simulink model "pcc_backstepping_piston_velocity_loop"  (R2021a)
settings: Solver=VariableStepAuto  StartTime=0.0  StopTime=70  MaxStep=0.001  RelTol=1e-3
undefined symbols (not defined in the file): l, q_eq, tol_q_stable
libraries: simulink_extras x4, simulink x3, pid_lib x1
settings Model: PauseTimes=0  Creator=maximilianstoelzle  LastModifiedBy=mstolzle
settings RTWCC: BuildConfiguration=Faster Runs

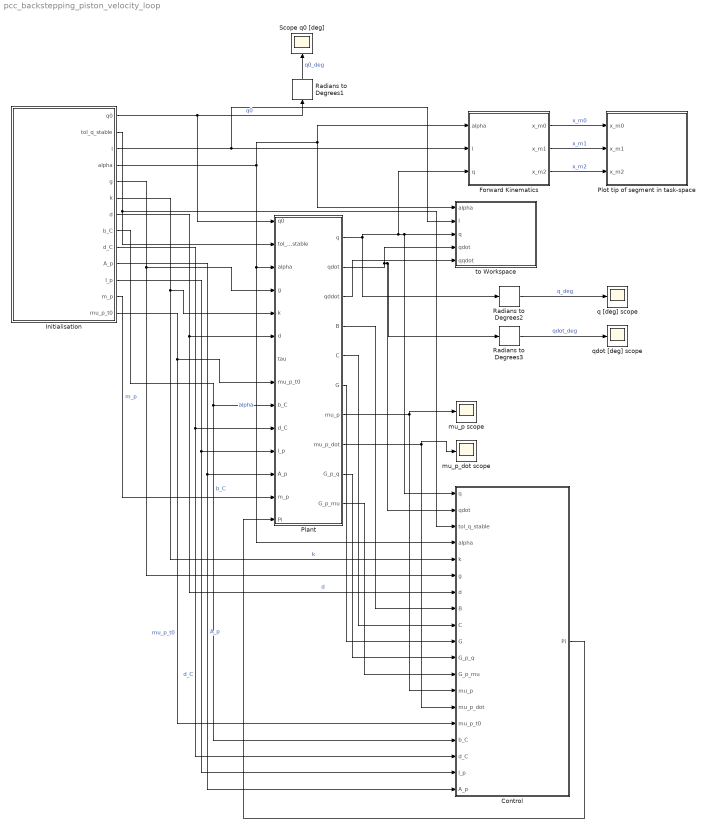
== system pcc_backstepping_piston_velocity_loop ==
  Control : Subsystem
  Forward Kinematics : MATLAB Function  TreatAsAtomicUnit=on
  Initialisation : Subsystem
  Plant : Subsystem
  Plot tip of segment in task-space : Subsystem
  Radians to Degrees1 : simulink_extras/Transformations/Radians to Degrees
  Radians to Degrees2 : simulink_extras/Transformations/Radians to Degrees
  Radians to Degrees3 : simulink_extras/Transformations/Radians to Degrees
  Scope q0 [deg] : Scope
  mu_p scope : Scope
  mu_p_dot scope : Scope
  q [deg] scope : Scope
  qdot [deg] scope : Scope
  to Workspace : Subsystem
  wires:
  Initialisation/12(m_p) -> Plant/13(m_p)  "m_p"
  Plant/5(C) -> Control/9(C)
  Initialisation/13(mu_p_t0) -> Control/15(mu_p_t0), Plant/8(mu_p_t0)  "mu_p_t0"
  Plant/10(G_p_mu) -> Control/12(G_p_mu)
  Initialisation/6(k) -> Control/5(k), Plant/5(k)  "k"
  Plant/8(mu_p_dot) -> mu_p_dot scope/1, Control/14(mu_p_dot)
  Plant/9(G_p_q) -> Control/11(G_p_q)
  Control/1(Pi) -> Plant/14(Pi)
  Radians to Degrees1/1 -> Scope q0 [deg]/1  "q0_deg"
  Plant/6(G) -> Control/10(G)
  Plant/4(B) -> Control/8(B)
  Initialisation/5(g) -> Control/6(g), Plant/4(g)
  Plant/3(qddot) -> to Workspace/5(qqdot)
  Radians to Degrees3/1 -> qdot [deg] scope/1  "qdot_deg"
  Forward Kinematics/3(x_m2) -> Plot tip of segment in task-space/3(x_m2)  "x_m2"
  Forward Kinematics/2(x_m1) -> Plot tip of segment in task-space/2(x_m1)  "x_m1"
  Forward Kinematics/1(x_m0) -> Plot tip of segment in task-space/1(x_m0)  "x_m0"
  Radians to Degrees2/1 -> q [deg] scope/1  "q_deg"
  Plant/7(mu_p) -> mu_p scope/1, Control/13(mu_p)
  Initialisation/11(l_p) -> Control/18(l_p), Plant/11(l_p)
  Initialisation/8(b_C) -> Control/16(b_C), Plant/9(b_C)  "b_C"
  Initialisation/9(d_C) -> Control/17(d_C), Plant/10(d_C)  "d_C"
  Initialisation/10(A_p) -> Control/19(A_p), Plant/12(A_p)  "A_p"
  Initialisation/1(q0) -> Plant/1(q0), Radians to Degrees1/1  "q0"
  Plant/1(q) -> Control/1(q), to Workspace/3(q), Forward Kinematics/3(q), Radians to Degrees2/1
  Plant/2(qdot) -> Control/2(qdot), Radians to Degrees3/1, to Workspace/4(qdot)
  Initialisation/7(d) -> Control/7(d), Plant/6(d)  "d"
  Initialisation/4(alpha) -> to Workspace/1(alpha), Forward Kinematics/1(alpha), Control/4(alpha), Plant/3(alpha)  "alpha"
  Initialisation/3(l) -> to Workspace/2(l), Forward Kinematics/2(l)
  Initialisation/2(tol_q_stable) -> Plant/2(tol_q_stable), Control/3(tol_q_stable)

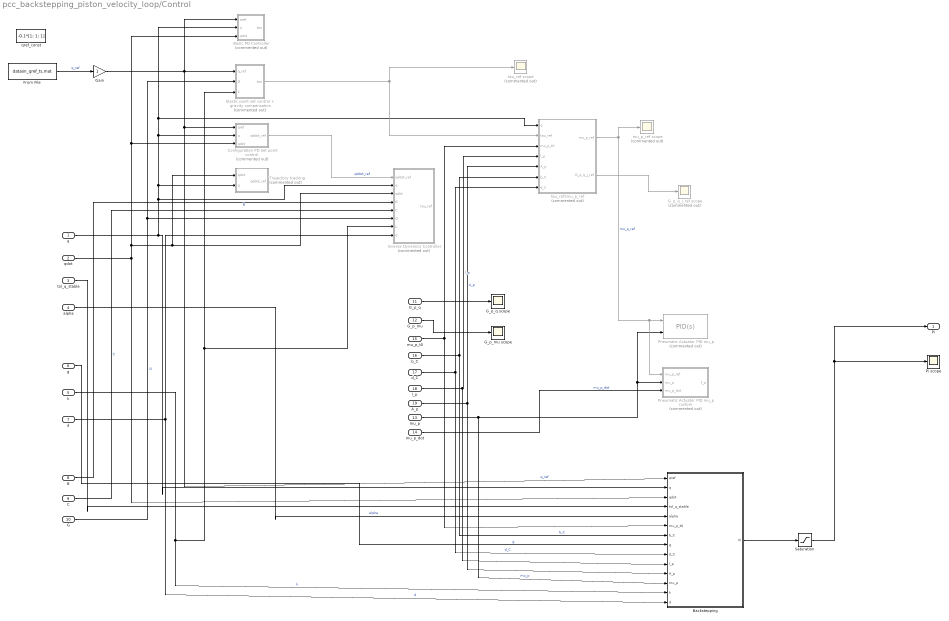
== system pcc_backstepping_piston_velocity_loop/Control ==
  q : Inport
  qdot : Inport  Port=2
  tol_q_stable : Inport  Port=3
  alpha : Inport  Port=4
  k : Inport  Port=5
  g : Inport  Port=6
  d : Inport  Port=7
  B : Inport  Port=8
  C : Inport  Port=9
  G : Inport  Port=10
  G_p_q : Inport  Port=11
  G_p_mu : Inport  Port=12
  mu_p : Inport  Port=13
  mu_p_dot : Inport  Port=14
  mu_p_t0 : Inport  Port=15
  b_C : Inport  Port=16
  d_C : Inport  Port=17
  l_p : Inport  Port=18
  A_p : Inport  Port=19
  Backstepping : Subsystem
  Basic PD Controller : Subsystem  Commented=on
  Configuration PD Set point control : Subsystem  Commented=on
  Elastic point set control + gravity compensation : MATLAB Function  Commented=on  TreatAsAtomicUnit=on
  From File : FromFile  FileName=data\in_qref_ts.mat  SampleTime=0  InterpolationWithinTimeRange=Zero order hold
  G_p_mu scope : Scope
  G_p_q scope : Scope
  G_p_q_j_ref scope : Scope  Commented=on
  Gain : Gain
  Inverse Dynamics Controller : MATLAB Function  Commented=on  TreatAsAtomicUnit=on
  Pi scope : Scope
  Pneumatic Actuator PID mu_p : pid_lib/PID Controller (2DOF)  Commented=on  Controller=PID  Form=Parallel  TimeDomain=Continuous-time  UseExternalTs=off  SampleTime=-1  IntegratorMethod=Forward Euler  FilterMethod=Forward Euler  ControllerParametersSource=internal  P=-3000  I=-500  D=-100  UseFilter=on  N=100  b=1  c=1  TunerSelectOption=Frequency Response Based  InitialConditionSource=internal  InitialConditionForIntegrator=0  InitialConditionForFilter=0  DifferentiatorICPrevScaledInput=0  ExternalReset=none  TrackingMode=off  Kt=1  LimitOutput=off  SatLimitsSource=internal  UpperSaturationLimit=inf  LowerSaturationLimit=-inf  LinearizeAsGain=on  AntiWindupMode=none  Kb=1  POutMin=[]  POutMax=[]  IOutMin=[]  IOutMax=[]  DOutMin=[]  DOutMax=[]  NOutMin=[]  NOutMax=[]  bOutMin=[]  bOutMax=[]  cOutMin=[]  cOutMax=[]  SumOutMin=[]  SumOutMax=[]  SaturationOutMin=[]  SaturationOutMax=[]  PParamMin=[]  PParamMax=[]  IParamMin=[]  IParamMax=[]  DParamMin=[]  DParamMax=[]  NParamMin=[]  NParamMax=[]  bParamMin=[]  bParamMax=[]  cParamMin=[]  cParamMax=[]  KbParamMin=[]  KbParamMax=[]  KtParamMin=[]  KtParamMax=[]  KbOutMin=[]  KbOutMax=[]  KtOutMin=[]  KtOutMax=[]  IntegratorOutMin=[]  IntegratorOutMax=[]  FilterOutMin=[]  FilterOutMax=[]  SumI1OutMin=[]  SumI1OutMax=[]  SumI2OutMin=[]  SumI2OutMax=[]  SumI3OutMin=[]  SumI3OutMax=[]  SumI4OutMin=[]  SumI4OutMax=[]  SumDOutMin=[]  SumDOutMax=[]  Sum1OutMin=[]  Sum1OutMax=[]  Sum2OutMin=[]  Sum2OutMax=[]  Sum3OutMin=[]  Sum3OutMax=[]  DifferentiatorOutMin=[]  DifferentiatorOutMax=[]  FilterDiffOutCoefMin=[]  FilterDiffOutCoefMax=[]  ReciprocalOutMin=[]  ReciprocalOutMax=[]  SumDenOutMin=[]  SumDenOutMax=[]  SumNumOutMin=[]  SumNumOutMax=[]  DivideOutMin=[]  DivideOutMax=[]  UdiffTsProdOutMin=[]  UdiffTsProdOutMax=[]  NTsProdOutMin=[]  NTsProdOutMax=[]  UintegralTsProdOutMin=[]  UintegralTsProdOutMax=[]  UngainTsProdOutMin=[]  UngainTsProdOutMax=[]  IntegratorContinuousStateAttributes=''  IntegratorStateMustResolveToSignalObject=off  IntegratorRTWStateStorageClass=Auto  FilterContinuousStateAttributes=''  FilterStateMustResolveToSignalObject=off  FilterRTWStateStorageClass=Auto  ParallelPVariant=InternalParameters  IdealPVariant=Disabled  IVariant=InternalParameters  DVariant=InternalParameters  bVariant=InternalParameters  cVariant=InternalParameters  IntegratorVariant=Continuous  SatVariant=Disabled  AWVariant=Passthrough  PCopyVariant=Disabled  TRVariant=Disabled  FdbkBlocksVariant=Forward  IdealPFdbkVariant=Disabled  SatFdbkVariant=Disabled  DerivativeFilterVariant=ContFilter  NVariant=InternalParameters  NCopyVariant=Disabled  FilterICVariant=InternalICsFilter  IntegratorICVariant=InternalICs  ExternalResetVariant=Disabled  TRSumVariant=Passthrough  SumFdbkVariant=Disabled  SumVariant=Sum_PID  TsampFilterVariant=InternalTs  TsampNgainVariant=Passthrough  TsampIntegralVariant=Passthrough  ExternalSaturationOutDataTypeStr=Inherit: Same as second input
      settings: SourceProductBaseCode=SL
  Pneumatic Actuator PID mu_p custom : Subsystem  Commented=on
  Saturation : Saturate  UpperLimit=1  LowerLimit=-1
  Trajectory tracking : Subsystem  Commented=on
  mu_p_ref scope : Scope  Commented=on
  qref_const : Constant  Value=-0.1*[1; 1; 1]
  tau_ref scope : Scope  Commented=on
  tau_ref2mu_p_ref : MATLAB Function  Commented=on  TreatAsAtomicUnit=on
  Pi : Outport
  wires:
  q/1 -> Inverse Dynamics Controller/2(q), Trajectory tracking/2(q), Configuration PD Set point control/2(q), tau_ref2mu_p_ref/1(q), Basic PD Controller/2(q), Backstepping/2(q)
  qdot/1 -> Backstepping/3(qdot), Basic PD Controller/3(qdot), Configuration PD Set point control/3(qdot), Trajectory tracking/1(qdot), Inverse Dynamics Controller/3(qdot)
  B/1 -> Inverse Dynamics Controller/4(B)  "B"
  C/1 -> Inverse Dynamics Controller/5(C)  "C"
  G/1 -> Elastic point set control + gravity compensation/2(G), Inverse Dynamics Controller/6(G)  "G"
  k/1 -> Backstepping/13(k), Elastic point set control + gravity compensation/3(k), Inverse Dynamics Controller/7(k)  "k"
  d/1 -> Inverse Dynamics Controller/8(d), Backstepping/14(d)  "d"
  Configuration PD Set point control/1(qddot_ref) -> Inverse Dynamics Controller/1(qddot_ref)  "qddot_ref"
  mu_p/1 -> Backstepping/12(mu_p), Pneumatic Actuator PID mu_p/2, Pneumatic Actuator PID mu_p custom/2(mu_p)  "mu_p"
  tau_ref2mu_p_ref/1(mu_p_ref) -> Pneumatic Actuator PID mu_p custom/1(mu_p_ref), Pneumatic Actuator PID mu_p/1, mu_p_ref scope/1  "mu_p_ref"
  mu_p_t0/1 -> tau_ref2mu_p_ref/3(mu_p_t0), Backstepping/6(mu_p_t0)
  b_C/1 -> Backstepping/7(b_C), tau_ref2mu_p_ref/6(b_C)  "b_C"
  d_C/1 -> Backstepping/9(d_C), tau_ref2mu_p_ref/7(d_C)  "d_C"
  l_p/1 -> Backstepping/10(l_p), tau_ref2mu_p_ref/4(l_p)  "l_p"
  A_p/1 -> tau_ref2mu_p_ref/5(A_p), Backstepping/11(A_p)  "A_p"
  tau_ref2mu_p_ref/2(G_p_q_j_ref) -> G_p_q_j_ref scope/1
  G_p_q/1 -> G_p_q scope/1
  G_p_mu/1 -> G_p_mu scope/1
  mu_p_dot/1 -> Pneumatic Actuator PID mu_p custom/3(mu_p_dot)  "mu_p_dot"
  alpha/1 -> Backstepping/5(alpha)  "alpha"
  g/1 -> Backstepping/8(g)  "g"
  Elastic point set control + gravity compensation/1(tau) -> tau_ref scope/1, tau_ref2mu_p_ref/2(tau_ref)
  Backstepping/1(Pi) -> Saturation/1
  Gain/1 -> Basic PD Controller/1(qref), Backstepping/1(qref), Configuration PD Set point control/1(qref), Elastic point set control + gravity compensation/1(q_ref)  "q_ref"
  From File/1 -> Gain/1  "q_ref"
  tol_q_stable/1 -> Backstepping/4(tol_q_stable)
  Saturation/1 -> Pi/1, Pi scope/1

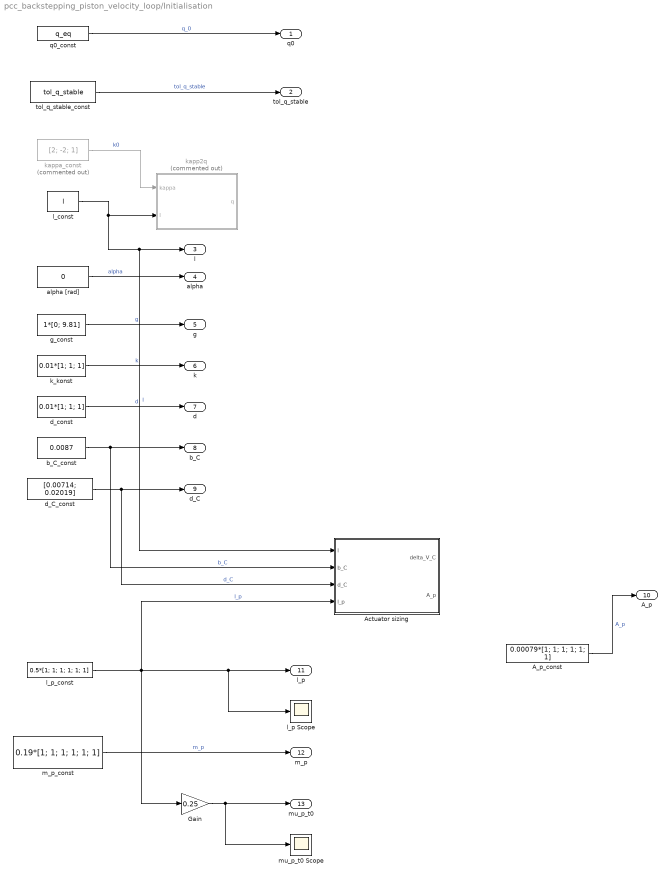
== system pcc_backstepping_piston_velocity_loop/Initialisation ==
  A_p_const : Constant  Value=0.00079*[1; 1; 1; 1; 1; 1]
  Actuator sizing : MATLAB Function  TreatAsAtomicUnit=on
  Gain : Gain  Gain=0.25
  alpha [rad] : Constant  Value=0
  b_C_const : Constant  Value=0.0087
  d_C_const : Constant  Value=[0.00714; 0.02019]
  d_const : Constant  Value=0.01*[1; 1; 1]
  g_const : Constant  Value=1*[0; 9.81]
  k_konst : Constant  Value=0.01*[1; 1; 1]
  kapp2q : MATLAB Function  Commented=on  TreatAsAtomicUnit=on
  kappa_const : Constant  Commented=on  Value=[2; -2; 1]
  l_const : Constant  Value=l
  l_p Scope : Scope
  l_p_const : Constant  Value=0.5*[1; 1; 1; 1; 1; 1]
  m_p_const : Constant  Value=0.19*[1; 1; 1; 1; 1; 1]
  mu_p_t0 Scope : Scope
  q0_const : Constant  Value=q_eq
  tol_q_stable_const : Constant  Value=tol_q_stable
  q0 : Outport
  tol_q_stable : Outport  Port=2
  l : Outport  Port=3
  alpha : Outport  Port=4
  g : Outport  Port=5
  k : Outport  Port=6
  d : Outport  Port=7
  b_C : Outport  Port=8
  d_C : Outport  Port=9
  A_p : Outport  Port=10
  l_p : Outport  Port=11
  m_p : Outport  Port=12
  mu_p_t0 : Outport  Port=13
  wires:
  kappa_const/1 -> kapp2q/1(kappa)  "k0"
  l_const/1 -> kapp2q/2(l), Actuator sizing/1(l), l/1  "l"
  alpha [rad]/1 -> alpha/1  "alpha"
  g_const/1 -> g/1  "g"
  k_konst/1 -> k/1  "k"
  d_C_const/1 -> Actuator sizing/3(d_C), d_C/1  "d_C"
  m_p_const/1 -> m_p/1  "m_p"
  b_C_const/1 -> Actuator sizing/2(b_C), b_C/1  "b_C"
  l_p_const/1 -> Gain/1, Actuator sizing/4(l_p), l_p Scope/1, l_p/1  "l_p"
  Gain/1 -> mu_p_t0 Scope/1, mu_p_t0/1
  d_const/1 -> d/1  "d"
  A_p_const/1 -> A_p/1  "A_p"
  q0_const/1 -> q0/1  "q_0"
  tol_q_stable_const/1 -> tol_q_stable/1  "tol_q_stable"

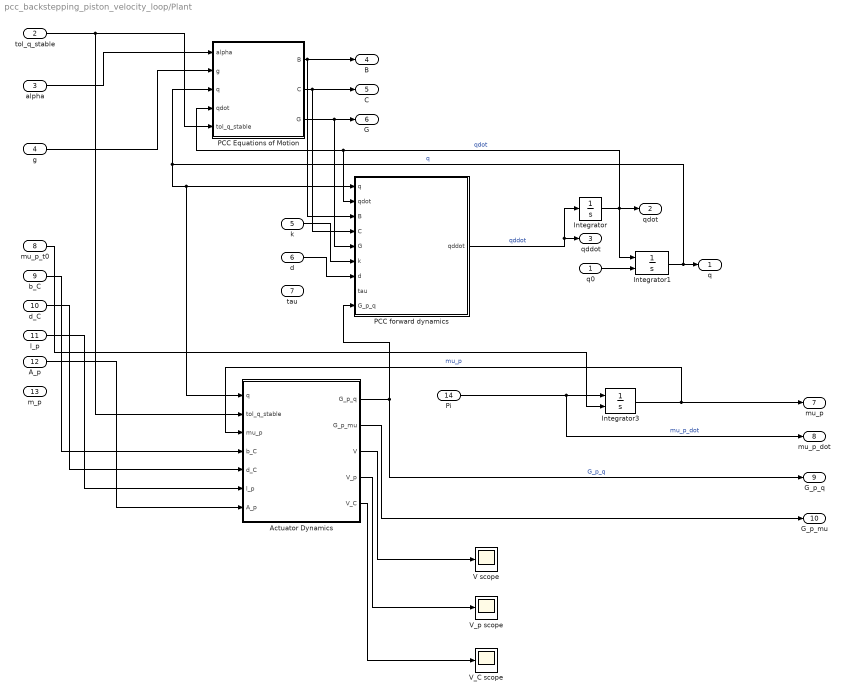
== system pcc_backstepping_piston_velocity_loop/Plant ==
  q0 : Inport
  tol_q_stable : Inport  Port=2
  alpha : Inport  Port=3
  g : Inport  Port=4
  k : Inport  Port=5
  d : Inport  Port=6
  tau : Inport  Port=7
  mu_p_t0 : Inport  Port=8
  b_C : Inport  Port=9
  d_C : Inport  Port=10
  l_p : Inport  Port=11
  A_p : Inport  Port=12
  m_p : Inport  Port=13
  Pi : Inport  Port=14
  Actuator Dynamics : MATLAB Function  TreatAsAtomicUnit=on
  Integrator : Integrator  InitialCondition=[0; 0; 0]
  Integrator1 : Integrator  InitialConditionSource=external
  Integrator3 : Integrator  InitialConditionSource=external  LowerSaturationLimit=[0; 0; 0; 0; 0; 0]
  PCC Equations of Motion : MATLAB Function  TreatAsAtomicUnit=on
  PCC forward dynamics : MATLAB Function  TreatAsAtomicUnit=on
  V scope : Scope
  V_C scope : Scope
  V_p scope : Scope
  q : Outport
  qdot : Outport  Port=2
  qddot : Outport  Port=3
  B : Outport  Port=4
  C : Outport  Port=5
  G : Outport  Port=6
  mu_p : Outport  Port=7
  mu_p_dot : Outport  Port=8
  G_p_q : Outport  Port=9
  G_p_mu : Outport  Port=10
  wires:
  g/1 -> PCC Equations of Motion/2(g)
  alpha/1 -> PCC Equations of Motion/1(alpha)
  q0/1 -> Integrator1/2
  k/1 -> PCC forward dynamics/6(k)
  PCC Equations of Motion/3(G) -> PCC forward dynamics/5(G), G/1
  PCC Equations of Motion/1(B) -> PCC forward dynamics/3(B), B/1
  Integrator1/1 -> PCC Equations of Motion/3(q), Actuator Dynamics/1(q), PCC forward dynamics/1(q), q/1  "q"
  PCC forward dynamics/1(qddot) -> Integrator/1, qddot/1  "qddot"
  d/1 -> PCC forward dynamics/7(d)
  Integrator/1 -> PCC forward dynamics/2(qdot), PCC Equations of Motion/4(qdot), Integrator1/1, qdot/1  "qdot"
  PCC Equations of Motion/2(C) -> PCC forward dynamics/4(C), C/1
  A_p/1 -> Actuator Dynamics/7(A_p)
  d_C/1 -> Actuator Dynamics/5(d_C)
  Pi/1 -> mu_p_dot/1, Integrator3/1  "mu_p_dot"
  b_C/1 -> Actuator Dynamics/4(b_C)
  l_p/1 -> Actuator Dynamics/6(l_p)
  Integrator3/1 -> Actuator Dynamics/3(mu_p), mu_p/1  "mu_p"
  Actuator Dynamics/1(G_p_q) -> G_p_q/1, PCC forward dynamics/9(G_p_q)  "G_p_q"
  Actuator Dynamics/2(G_p_mu) -> G_p_mu/1
  mu_p_t0/1 -> Integrator3/2
  Actuator Dynamics/3(V) -> V scope/1
  Actuator Dynamics/5(V_C) -> V_C scope/1
  Actuator Dynamics/4(V_p) -> V_p scope/1
  tol_q_stable/1 -> PCC Equations of Motion/5(tol_q_stable), Actuator Dynamics/2(tol_q_stable)

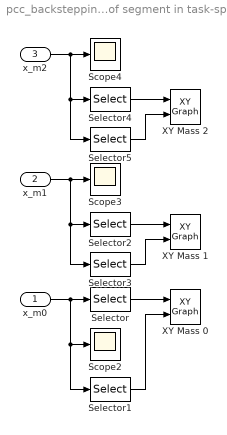
== system pcc_backstepping_piston_velocity_loop/Plot tip of segment in task-space ==
  x_m0 : Inport
  x_m1 : Inport  Port=2
  x_m2 : Inport  Port=3
  Scope2 : Scope
  Scope3 : Scope
  Scope4 : Scope
  Selector : Selector  InputPortWidth=2  IndexOptions=Index vector (dialog)  Indices=[1]  OutputSizes=1
  Selector1 : Selector  InputPortWidth=2  IndexOptions=Index vector (dialog)  Indices=[2]  OutputSizes=1
  Selector2 : Selector  InputPortWidth=2  IndexOptions=Index vector (dialog)  Indices=[1]  OutputSizes=1
  Selector3 : Selector  InputPortWidth=2  IndexOptions=Index vector (dialog)  Indices=[2]  OutputSizes=1
  Selector4 : Selector  InputPortWidth=2  IndexOptions=Index vector (dialog)  Indices=[1]  OutputSizes=1
  Selector5 : Selector  InputPortWidth=2  IndexOptions=Index vector (dialog)  Indices=[2]  OutputSizes=1
  XY Mass 0 : simulink/Sinks/XY Graph  xmin=-1.2*sum(l)  xmax=1.2*sum(l)  ymin=-1.2*sum(l)  ymax=1.2*sum(l)  st=-1
  XY Mass 1 : simulink/Sinks/XY Graph  xmin=-1.2*sum(l)  xmax=1.2*sum(l)  ymin=-1.2*sum(l)  ymax=1.2*sum(l)  st=-1
  XY Mass 2 : simulink/Sinks/XY Graph  xmin=-1.2*sum(l)  xmax=1.2*sum(l)  ymin=-1.2*sum(l)  ymax=1.2*sum(l)  st=-1
  wires:
  x_m2/1 -> Selector5/1, Selector4/1, Scope4/1
  Selector/1 -> XY Mass 0/1
  x_m1/1 -> Selector3/1, Selector2/1, Scope3/1
  Selector5/1 -> XY Mass 2/2
  Selector3/1 -> XY Mass 1/2
  Selector1/1 -> XY Mass 0/2
  x_m0/1 -> Scope2/1, Selector1/1, Selector/1
  Selector4/1 -> XY Mass 2/1
  Selector2/1 -> XY Mass 1/1

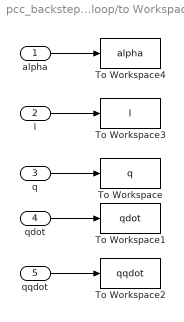
== system pcc_backstepping_piston_velocity_loop/to Workspace ==
  alpha : Inport
  l : Inport  Port=2
  q : Inport  Port=3
  qdot : Inport  Port=4
  qqdot : Inport  Port=5
  To Workspace : ToWorkspace  VariableName=q  SaveFormat=Timeseries  SampleTime=-1
  To Workspace1 : ToWorkspace  VariableName=qdot  SaveFormat=Timeseries  SampleTime=-1
  To Workspace2 : ToWorkspace  VariableName=qqdot  SaveFormat=Timeseries  SampleTime=-1
  To Workspace3 : ToWorkspace  VariableName=l  SaveFormat=Timeseries  SampleTime=-1
  To Workspace4 : ToWorkspace  VariableName=alpha  SaveFormat=Timeseries  SampleTime=-1
  wires:
  alpha/1 -> To Workspace4/1
  qdot/1 -> To Workspace1/1
  l/1 -> To Workspace3/1
  qqdot/1 -> To Workspace2/1
  q/1 -> To Workspace/1

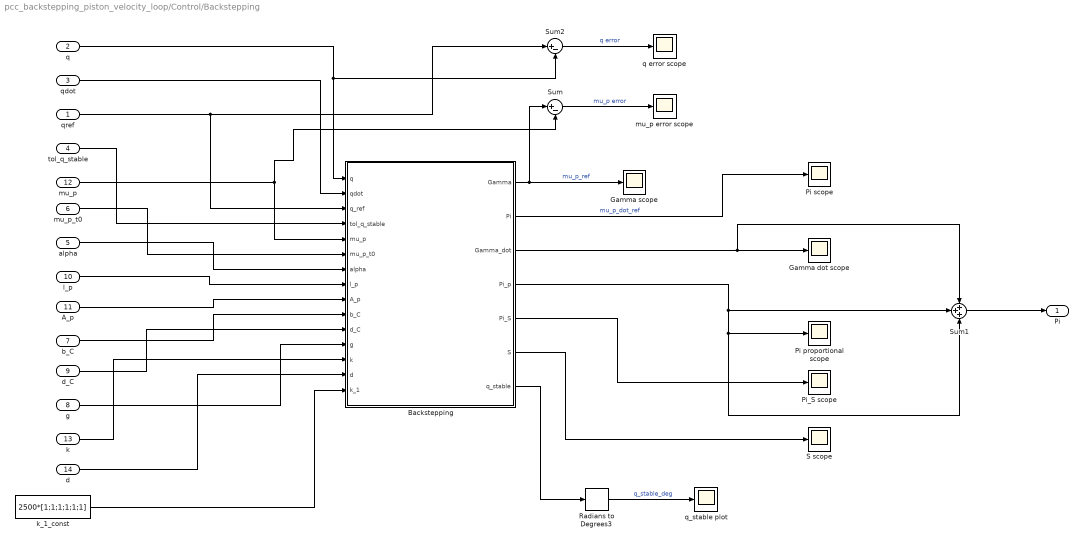
== system pcc_backstepping_piston_velocity_loop/Control/Backstepping ==
  qref : Inport
  q : Inport  Port=2
  qdot : Inport  Port=3
  tol_q_stable : Inport  Port=4
  alpha : Inport  Port=5
  mu_p_t0 : Inport  Port=6
  b_C : Inport  Port=7
  g : Inport  Port=8
  d_C : Inport  Port=9
  l_p : Inport  Port=10
  A_p : Inport  Port=11
  mu_p : Inport  Port=12
  k : Inport  Port=13
  d : Inport  Port=14
  Backstepping : MATLAB Function  TreatAsAtomicUnit=on
  Gamma dot scope : Scope
  Gamma scope : Scope
  Pi proportional scope : Scope
  Pi scope : Scope
  Pi_S scope : Scope
  Radians to Degrees3 : simulink_extras/Transformations/Radians to Degrees
  S scope : Scope
  Sum : Sum  Inputs=|+-
  Sum1 : Sum  Inputs=+++
  Sum2 : Sum  Inputs=|+-
  k_1_const : Constant  Value=2500*[1;1;1;1;1;1]
  mu_p error scope : Scope
  q error scope : Scope
  q_stable plot : Scope
  Pi : Outport
  wires:
  mu_p/1 -> Sum/2, Backstepping/5(mu_p)
  k_1_const/1 -> Backstepping/15(k_1)
  qref/1 -> Backstepping/3(q_ref), Sum2/1
  q/1 -> Sum2/2, Backstepping/1(q)
  Backstepping/2(Pi) -> Pi scope/1  "mu_p_dot_ref"
  Backstepping/1(Gamma) -> Gamma scope/1, Sum/1  "mu_p_ref"
  qdot/1 -> Backstepping/2(qdot)
  A_p/1 -> Backstepping/9(A_p)
  k/1 -> Backstepping/13(k)
  alpha/1 -> Backstepping/7(alpha)
  b_C/1 -> Backstepping/10(b_C)
  d_C/1 -> Backstepping/11(d_C)
  g/1 -> Backstepping/12(g)
  d/1 -> Backstepping/14(d)
  l_p/1 -> Backstepping/8(l_p)
  mu_p_t0/1 -> Backstepping/6(mu_p_t0)
  Sum/1 -> mu_p error scope/1  "mu_p error"
  Backstepping/4(Pi_p) -> Sum1/3, Pi proportional scope/1, Sum1/2
  Backstepping/5(Pi_S) -> Pi_S scope/1
  Sum1/1 -> Pi/1
  Backstepping/6(S) -> S scope/1
  Backstepping/3(Gamma_dot) -> Sum1/1, Gamma dot scope/1
  tol_q_stable/1 -> Backstepping/4(tol_q_stable)
  Backstepping/7(q_stable) -> Radians to Degrees3/1
  Radians to Degrees3/1 -> q_stable plot/1  "q_stable_deg"
  Sum2/1 -> q error scope/1  "q error"

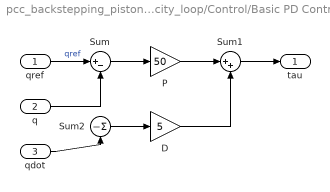
== system pcc_backstepping_piston_velocity_loop/Control/Basic PD Controller ==
  qref : Inport
  q : Inport  Port=2
  qdot : Inport  Port=3
  D : Gain  Gain=5
  P : Gain  Gain=50
  Sum : Sum  Inputs=|+-
  Sum1 : Sum  Inputs=|++
  Sum2 : Sum  Inputs=||-
  tau : Outport
  wires:
  qdot/1 -> Sum2/1
  Sum1/1 -> tau/1
  D/1 -> Sum1/2
  q/1 -> Sum/2
  qref/1 -> Sum/1  "qref"
  Sum/1 -> P/1
  P/1 -> Sum1/1
  Sum2/1 -> D/1

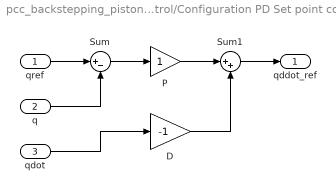
== system pcc_backstepping_piston_velocity_loop/Control/Configuration PD Set point control ==
  qref : Inport
  q : Inport  Port=2
  qdot : Inport  Port=3
  D : Gain  Gain=-1
  P : Gain
  Sum : Sum  Inputs=|+-
  Sum1 : Sum  Inputs=|++
  qddot_ref : Outport
  wires:
  Sum1/1 -> qddot_ref/1
  D/1 -> Sum1/2
  q/1 -> Sum/2
  qref/1 -> Sum/1
  Sum/1 -> P/1
  P/1 -> Sum1/1
  qdot/1 -> D/1

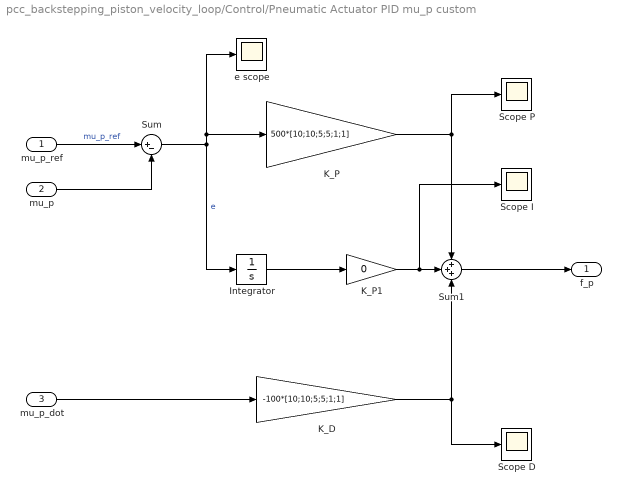
== system pcc_backstepping_piston_velocity_loop/Control/Pneumatic Actuator PID mu_p custom ==
  mu_p_ref : Inport
  mu_p : Inport  Port=2
  mu_p_dot : Inport  Port=3
  Integrator : Integrator
  K_D : Gain  Gain=-100*[10;10;5;5;1;1]
  K_P : Gain  Gain=500*[10;10;5;5;1;1]
  K_P1 : Gain  Gain=0
  Scope D : Scope
  Scope I : Scope
  Scope P : Scope
  Sum : Sum  Inputs=|+-
  Sum1 : Sum  Inputs=+++
  e scope : Scope
  f_p : Outport
  wires:
  Sum1/1 -> f_p/1
  K_D/1 -> Sum1/3, Scope D/1
  mu_p/1 -> Sum/2
  mu_p_ref/1 -> Sum/1  "mu_p_ref"
  Sum/1 -> e scope/1, K_P/1, Integrator/1  "e"
  K_P/1 -> Scope P/1, Sum1/1
  mu_p_dot/1 -> K_D/1
  Integrator/1 -> K_P1/1
  K_P1/1 -> Sum1/2, Scope I/1

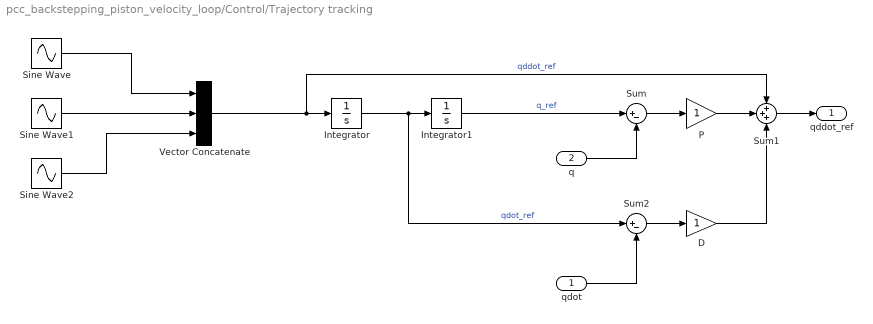
== system pcc_backstepping_piston_velocity_loop/Control/Trajectory tracking ==
  qdot : Inport
  q : Inport  Port=2
  D : Gain
  Integrator : Integrator  InitialCondition=[-0.25, -0.5, -1]
  Integrator1 : Integrator
  P : Gain
  Sine Wave : Sin  Amplitude=0.25  Samples=100  SampleTime=0
  Sine Wave1 : Sin  Amplitude=0.5  SampleTime=0
  Sine Wave2 : Sin  SampleTime=0
  Sum : Sum  Inputs=|+-
  Sum1 : Sum  Inputs=+++
  Sum2 : Sum  Inputs=|+-
  Vector Concatenate : Concatenate  NumInputs=3
  qddot_ref : Outport
  wires:
  Sum1/1 -> qddot_ref/1
  q/1 -> Sum/2
  Sum/1 -> P/1
  Vector Concatenate/1 -> Sum1/1, Integrator/1  "qddot_ref"
  Integrator/1 -> Sum2/1, Integrator1/1  "qdot_ref"
  Integrator1/1 -> Sum/1  "q_ref"
  qdot/1 -> Sum2/2
  Sum2/1 -> D/1
  D/1 -> Sum1/3
  P/1 -> Sum1/2
  Sine Wave/1 -> Vector Concatenate/1
  Sine Wave1/1 -> Vector Concatenate/2
  Sine Wave2/1 -> Vector Concatenate/3

== matlab function pcc_backstepping_piston_velocity_loop/Control/Elastic point set control + gravity compensation ==
  data: q_ref input; tau output; G input; k input
function tau = fcn(q_ref, G, k)
    tau = k.*q_ref + G;
end

== matlab function pcc_backstepping_piston_velocity_loop/Plant/Actuator Dynamics ==
  data: q input; tol_q_stable input; mu_p input; b_C input; d_C input; l_p input; A_p input; G_p_q output; G_p_mu output; V output; V_p output; V_C output
function [G_p_q, G_p_mu, V, V_p, V_C]  = actuator_dynamics(q, tol_q_stable, mu_p, b_C, d_C, l_p, A_p)
    % introduce tolerance for numerical stability
    q_stable = set_min_abs_val(q, tol_q_stable);

    % volume of fluid
    V = V_fun(q_stable, mu_p, A_p, b_C, d_C);
    V_p = V_p_fun(mu_p, A_p);
    V_C = V_C_fun(q_stable, b_C, d_C);

    % potential forces by fluid
    G_p_q = G_p_q_fun(q_stable, mu_p, l_p, A_p, b_C, d_C);
    G_p_mu = G_p_mu_fun(q_stable, mu_p, l_p, A_p, b_C, d_C);
end

== matlab function pcc_backstepping_piston_velocity_loop/Initialisation/Actuator sizing ==
  data: l input; delta_V_C output; b_C input; d_C input; l_p input; A_p output
function [delta_V_C, A_p]= piston_sizing(l, b_C, d_C, l_p)
    q_min = -90/180*pi*ones(length(l), 1);
    q_max = 90/180*pi*ones(length(l), 1);
    delta_V_C = abs(V_C_fun(q_max, b_C, d_C) - V_C_fun(q_min, b_C, d_C));
    A_p = 1*delta_V_C ./ l_p;
end

== matlab function pcc_backstepping_piston_velocity_loop/Control/tau_ref2mu_p_ref ==
  data: q input; tau_ref input; mu_p_ref output; mu_p_t0 input; l_p input; A_p input; b_C input; d_C input; G_p_q_j_ref output
function [mu_p_ref, G_p_q_j_ref]= tau_ref2mu_p_ref(q, tau_ref, mu_p_t0, l_p, A_p, b_C, d_C)
    mu_p_ref = mu_p_ref_fun(q, tau_ref, mu_p_t0, l_p, A_p, b_C, d_C);
    G_p_q_j_ref = G_p_q_j_ref_fun(tau_ref, mu_p_t0, l_p, A_p, b_C, d_C);
end

== matlab function pcc_backstepping_piston_velocity_loop/Control/Backstepping/Backstepping ==
  data: Gamma output; Pi output; q input; qdot input; q_ref input; tol_q_stable input; mu_p input; mu_p_t0 input; alpha input; l_p input; A_p input; b_C input; d_C input; g input; k input; d input; k_1 input; Gamma_dot output; Pi_p output; Pi_S output; S output; q_stable output
function [Gamma, Pi, Gamma_dot, Pi_p, Pi_S, S, q_stable]= Pi_fun(...
          q, qdot, q_ref, tol_q_stable, mu_p, mu_p_t0, ...
          alpha, l_p, A_p, b_C, d_C, g, k, d, k_1)
    % introduce tolerance for numerical stability
    q_stable = set_min_abs_val(q, tol_q_stable);
    q_stable_gamma_dot = set_min_abs_val(q, tol_q_stable*2);
      
    % Proportional gain for approaching the desired piston position
    K_1 = diag(k_1);
    
    % Components of equations of motion
    B = B_fun(q_stable);
%     B_dot = B_dot_fun(q, qdot);
%     C = C_fun(q, qdot);
%     G = G_fun(q, alpha, g);
    
    % potential forces by fluid
%     G_p_q = G_p_q_fun(q, mu_p, l_p, A_p, b_C, d_C);
%     G_p_mu = G_p_mu_fun(q, mu_p, l_p, A_p, b_C, d_C);
    
    % acceleration of system
%     qddot = -B^(-1)*(C*qdot + G + k.*q + d.*qdot + G_p_q);
    
    % Lyapunov function H
    dH_spc_dqdot = dH_spc_dqdot_fun(q_stable, qdot, alpha);
%     dH_spc_dqdot_dot = dH_spc_dqdot_dot_fun(q, qdot, qddot);

    % Gamma
    Gamma = Gamma_fun(q_stable, q_ref, mu_p_t0, alpha, l_p, A_p, b_C, d_C, g, k);
%     dGamma_dq = dGamma_dq_fun(q, q_ref, mu_p_t0, alpha, l_p, A_p, b_C, d_C, g, k);
    Gamma_dot = Gamma_dot_fun(q_stable_gamma_dot, qdot, q_ref, mu_p_t0, alpha, l_p, A_p, b_C, d_C, g, k);
    % dGamma_dot_dq = dGamma_dot_dq_fun(q, qdot, q_ref, mu_p_t0, alpha, l_p, A_p, b_C, d_C, g, k);
    
    % Lemma 
    S = S_fun(q_stable, q_ref, mu_p, mu_p_t0, alpha, l_p, A_p, b_C, d_C, g, k);
%     S_dot = S_dot_fun(q, qdot, q_ref, mu_p, mu_p_t0, alpha, l_p, A_p, b_C, d_C, g, k);
    
    % Pi = Gamma_dot + K_1*(mu_p - Gamma) - S'*(B^(-1))'*dH_spc_dqdot';
    Pi_p = - K_1*(mu_p - Gamma);
    Pi_S = S'*(B^(-1))'*dH_spc_dqdot';
    Pi = Gamma_dot + Pi_p + Pi_S;
    
%     Pi_dot = dGamma_dot_dq*qdot + dGamma_dq*qddot ...
%              - K_1*dGamma_dq*qdot ...
%              - S_dot'*(B^(-1))'*dH_spc_dqdot' ...
%              + S'*(B^(-1)*B_dot*B^(-1))'*dH_spc_dqdot' ...
%              - S'*(B^(-1))'*dH_spc_dqdot_dot;
    
%     Psi = G_p_mu + Pi_dot + K_2*(mu_p_dot-Pi) - (mu_p-Gamma);
end

== matlab function pcc_backstepping_piston_velocity_loop/Forward Kinematics ==
  data: alpha input; l input; x_m0 output; q input; x_m1 output; x_m2 output
function [x_m0, x_m1, x_m2] = forward_kinematics(alpha, l, q)
    % introduce tolerance for numerical stability
    q = set_min_abs_val(q, 0.005);

    x_m0 = q2x0_fun(l(1), q, alpha);
    x_m1 = q2x1_fun(l(2), q, alpha);
    x_m2 = q2x2_fun(l(3), q, alpha);
end

== matlab function pcc_backstepping_piston_velocity_loop/Plant/PCC forward dynamics ==
  data: q input; qdot input; B input; qddot output; C input; G input; k input; d input; tau input; G_p_q input
function qddot  = pcc_forward_dynamics(q, qdot, B, C, G, k, d, tau, G_p_q)
   qddot = B^(-1)*(-(C*qdot)-G-(k.*q)-(d.*qdot)-G_p_q+tau);
end

== matlab function pcc_backstepping_piston_velocity_loop/Initialisation/kapp2q ==
  data: kappa input; q output; l input
function q = kappa2q(kappa, l)
    q = [kappa(1) * l(1);
         kappa(2) * l(2);
         kappa(3) * l(3)];
end

== matlab function pcc_backstepping_piston_velocity_loop/Plant/PCC Equations of Motion ==
  data: alpha input; B output; g input; q input; qdot input; C output; G output; tol_q_stable input
function [B, C, G]  = pcc_eom(alpha, g, q, qdot, tol_q_stable)
    % introduce tolerance for numerical stability
    q_stable = set_min_abs_val(q, tol_q_stable);
    
    B = B_fun(q_stable);
    
    C = C_fun(q_stable, qdot);
    
    G = G_fun(q_stable, alpha, g);
end

== matlab function pcc_backstepping_piston_velocity_loop/Control/Inverse Dynamics Controller ==
  data: qddot_ref input; q input; tau_ref output; qdot input; B input; C input; G input; k input; d input
function tau_ref = fcn(qddot_ref, q, qdot, B, C, G, k, d)
    tau_ref = B*qddot_ref + C*qdot + G + k.*q + d.*qdot;
end
